simulink model "invertor_control"  (R2017a)
settings: Solver=VariableStepAuto  StartTime=0.0  StopTime=0.1  RelTol=1e-3
libraries: simulink x8, powerlib_meascontrol x3, dspsrcs4 x1
settings Model: Creator=VV  LastModifiedBy=VV

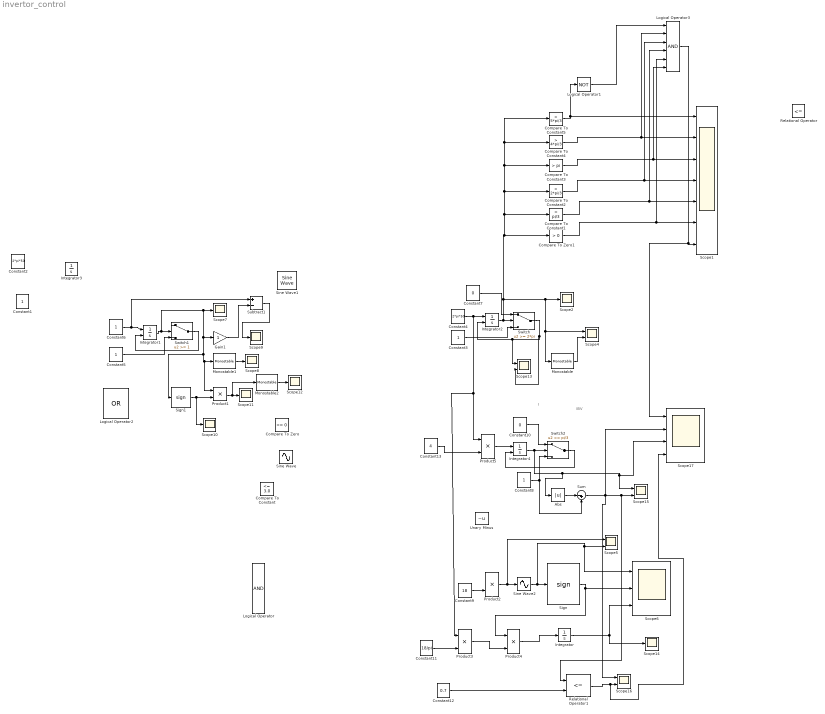
== system invertor_control ==
  note: IBV
  note: I
  Abs : Abs
  Compare To Constant : simulink/Logic and Bit Operations/Compare To Constant  relop=<=  const=3.0  OutDataTypeStr=boolean
  Compare To Constant1 : simulink/Logic and Bit Operations/Compare To Constant  relop=>  const=pi/3  OutDataTypeStr=boolean
  Compare To Constant2 : simulink/Logic and Bit Operations/Compare To Constant  relop=>  const=2*pi/3  OutDataTypeStr=boolean
  Compare To Constant3 : simulink/Logic and Bit Operations/Compare To Constant  relop=>  const=pi  OutDataTypeStr=boolean
  Compare To Constant4 : simulink/Logic and Bit Operations/Compare To Constant  relop=>  const=4*pi/3  OutDataTypeStr=boolean
  Compare To Constant5 : simulink/Logic and Bit Operations/Compare To Constant  relop=>  const=5*pi/3  OutDataTypeStr=boolean
  Compare To Zero : simulink/Logic and Bit Operations/Compare To Zero  relop=<=  OutDataTypeStr=boolean
  Compare To Zero1 : simulink/Logic and Bit Operations/Compare To Zero  relop=>  OutDataTypeStr=boolean
  Constant{1,3,5..6,8} (5 alike) : Constant  VectorParams1D=off  OutDataTypeStr=double
  Constant10 : Constant  Value=0  VectorParams1D=off  OutDataTypeStr=double
  Constant11 : Constant  Value=18/pi  VectorParams1D=off  OutDataTypeStr=double
  Constant12 : Constant  Value=0.7  VectorParams1D=off  OutDataTypeStr=double
  Constant13 : Constant  Value=4  VectorParams1D=off  OutDataTypeStr=double
  Constant2 : Constant  Value=2*pi*50  VectorParams1D=off  OutDataTypeStr=double
  Constant4 : Constant  Value=2*pi*50  VectorParams1D=off  OutDataTypeStr=double
  Constant7 : Constant  Value=0  VectorParams1D=off  OutDataTypeStr=double
  Constant9 : Constant  Value=18  VectorParams1D=off  OutDataTypeStr=double
  Gain1 : Gain
  Integrator : Integrator
  Integrator1 : Integrator  ExternalReset=falling
  Integrator2 : Integrator  ExternalReset=falling
  Integrator3 : Integrator  ExternalReset=falling
  Integrator4 : Integrator  ExternalReset=falling  InitialCondition=-pi/3
  Logical Operator : Logic  Inputs=6  AllPortsSameDT=off  OutDataTypeStr=boolean
  Logical Operator1 : Logic  Operator=NOT  AllPortsSameDT=off  OutDataTypeStr=boolean
  Logical Operator2 : Logic  Operator=OR  Inputs=3  AllPortsSameDT=off  OutDataTypeStr=boolean
  Logical Operator3 : Logic  Inputs=6  AllPortsSameDT=off  OutDataTypeStr=boolean
  Monostable : powerlib_meascontrol/Logic/Monostable  EdgeDetect=Falling  PulseDuration=0.0001  ic=0  Ts=0
      settings: SourceProductName=Simscape Power Systems  SourceProductBaseCode=PS
  Monostable1 : powerlib_meascontrol/Logic/Monostable  EdgeDetect=Falling  PulseDuration=0.0001  ic=0  Ts=0
      settings: SourceProductName=Simscape Power Systems  SourceProductBaseCode=PS
  Monostable2 : powerlib_meascontrol/Logic/Monostable  EdgeDetect=Falling  PulseDuration=0.0001  ic=1  Ts=0
      settings: SourceProductName=Simscape Power Systems  SourceProductBaseCode=PS
  Product{1..5} (5 alike) : Product
  Relational Operator : RelationalOperator  Operator=<=  OutDataTypeStr=boolean  RndMeth=Simplest
  Relational Operator1 : RelationalOperator  Operator=<=  OutDataTypeStr=boolean  RndMeth=Simplest
  Scope1 : Scope  NumInputPorts=7
  Scope{2,7..12,14} (8 alike) : Scope
  Scope{4..5,13,15..16} (5 alike) : Scope  NumInputPorts=2
  Scope17 : Scope  NumInputPorts=4
  Scope6 : Scope  NumInputPorts=3
  Sign : Signum
  Sign1 : Signum
  Sine Wave : Sin  Amplitude=2  Frequency=pi*10  SampleTime=0
  Sine Wave1 : dspsrcs4/Sine Wave  Amplitude=1  Frequency=100  Phase=0  SampleMode=Discrete  OutComplex=Real  CompMethod=Trigonometric fcn  TableSize=Speed  SampleTime=1/1000  SamplesPerFrame=1  ResetState=Restart at time zero  OutputFrames=off  dataType=double  wordLen=16  udDataType=sfix(16)  fracBitsMode=Best precision  numFracBits=15  OutDataTypeStr=double  LastOutDataTypeStr=double
  Sine Wave2 : Sin  TimeSource=Use external signal  SampleTime=0
  Subtract1 : Sum  Inputs=+-
  Sum : Sum  Inputs=|-+
  Switch : Switch  Threshold=2*pi
  Switch1 : Switch  Threshold=1
  Switch2 : Switch  Threshold=pi/3
  Unary Minus : UnaryMinus
  wires:
  Gain1/1 -> Subtract1/2
  Constant7/1 -> Switch/1
  Monostable2/1 -> Scope12/1
  Switch/1 -> Scope13/1, Integrator2/2, Scope13/2
  Product1/1 -> Monostable2/1, Scope11/1
  Integrator2/1 -> Compare To Constant1/1, Compare To Constant2/1, Compare To Constant3/1, Compare To Constant4/1, Compare To Constant5/1, Compare To Zero1/1, Scope2/1, Scope4/1, Monostable/1, Switch/2
  Sign1/1 -> Product1/2, Scope10/1
  Constant3/1 -> Switch/3
  Switch1/1 -> Integrator1/2
  Monostable/1 -> Scope4/2
  Integrator1/1 -> Scope7/1, Gain1/1, Sign1/1, Monostable1/1, Product1/1, Switch1/2
  Constant5/1 -> Switch1/3
  Monostable1/1 -> Scope8/1
  Constant6/1 -> Subtract1/1, Integrator1/1
  Subtract1/1 -> Scope9/1
  Constant4/1 -> Product5/1, Product3/1, Integrator2/1
  Compare To Zero1/1 -> Logical Operator3/5, Scope1/6
  Compare To Constant1/1 -> Logical Operator3/4, Scope1/5
  Compare To Constant2/1 -> Logical Operator3/3, Scope1/4
  Compare To Constant3/1 -> Scope1/3, Logical Operator3/6
  Compare To Constant4/1 -> Logical Operator3/2, Scope1/2
  Compare To Constant5/1 -> Logical Operator1/1, Scope1/1
  Constant9/1 -> Product2/2
  Switch2/1 -> Integrator4/2
  Constant8/1 -> Switch2/3, Sum/2
  Integrator4/1 -> Abs/1, Scope17/3, Scope15/1, Switch2/2
  Constant10/1 -> Switch2/1
  Product2/1 -> Scope5/1, Sine Wave2/1
  Sine Wave2/1 -> Scope5/2, Scope6/1, Sign/1
  Sign/1 -> Product4/1, Scope6/2
  Integrator/1 -> Scope14/1, Scope6/3
  Product4/1 -> Integrator/1
  Constant11/1 -> Product3/2
  Product3/1 -> Product4/2
  Constant12/1 -> Relational Operator1/2
  Relational Operator1/1 -> Scope17/4, Scope16/2
  Logical Operator3/1 -> Scope17/1, Scope1/7
  Logical Operator1/1 -> Logical Operator3/1
  Product5/1 -> Integrator4/1
  Constant13/1 -> Product5/2
  Abs/1 -> Sum/1
  Sum/1 -> Scope16/1, Scope17/2, Relational Operator1/1, Scope15/2
